simulink model "lab1_1"  (R2021a)
settings: Solver=VariableStepAuto  StartTime=0.0  StopTime=30  RelTol=1e-10  AbsTol=1e-10
values from neighbouring files (symbols this model uses):
  den = cell2mat(den)    [lab1.m]
  den1 = cell2mat(den1)    [lab1.m]
  num = cell2mat(num)    [lab1.m]
  num1 = cell2mat(num1)    [lab1.m]
settings Model: Creator=markalex  LastModifiedBy=markalex

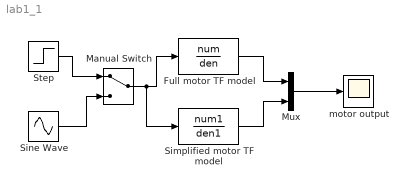
== system lab1_1 ==
  Full motor TF model : TransferFcn  Numerator=num  Denominator=den
  Manual Switch : ManualSwitch
  Mux : Mux  Inputs=2
  Simplified motor TF model : TransferFcn  Numerator=num1  Denominator=den1
  Sine Wave : Sin  SampleTime=0
  Step : Step  Time=0  SampleTime=0
  motor output : Scope
  wires:
  Sine Wave/1 -> Manual Switch/2
  Step/1 -> Manual Switch/1
  Manual Switch/1 -> Simplified motor TF model/1, Full motor TF model/1
  Full motor TF model/1 -> Mux/1
  Simplified motor TF model/1 -> Mux/2
  Mux/1 -> motor output/1
